simulink model "Comparison_between_Controllers"  (R2018b)
settings: Solver=VariableStepAuto  StartTime=0.0  StopTime=20000  FixedStep=1  RelTol=1e-3
undefined symbols (not defined in the file or in its folder): s
libraries: cstblocks x13, simulink x6, mpclib x3, slident x1
settings Model: Creator=Trips  LastModifiedBy=Trips

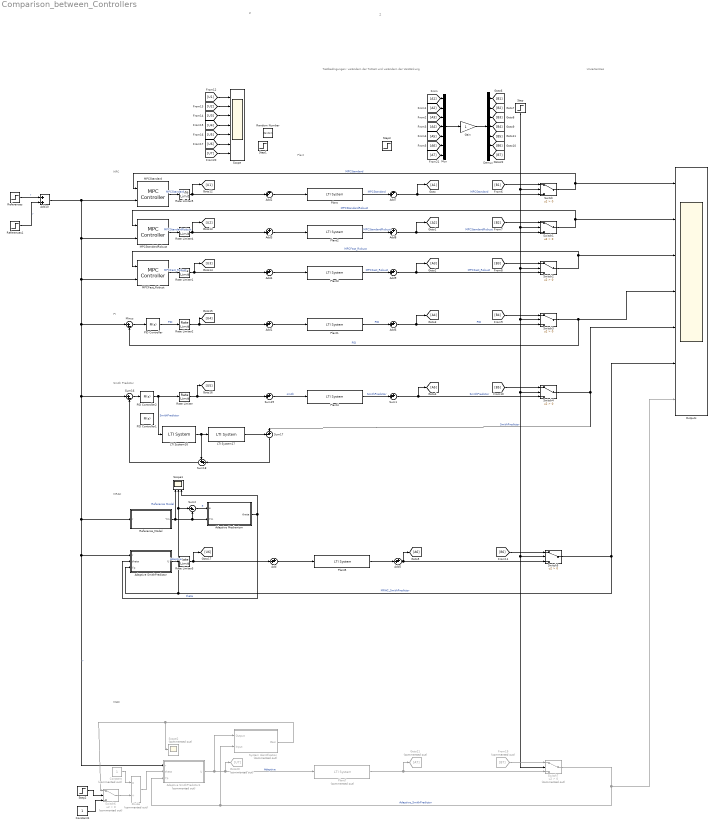
== system Comparison_between_Controllers ==
  note: MPC
  note: Testbedingungen: verändern der Totzeit und verändern der Verstärkung
  note: PI
  note: Smith Predictor
  note: Z
  note: Uncertainties
  note: Plant
  note: MRAC
  note: MIAC
  note: Z
  Adaptive Mechanism : Subsystem
  Adaptive SmithPredictor : Subsystem
  Adaptive SmithPredictor1 : Subsystem  Commented=on
  Add{,1..9} (10 alike) : Sum  Inputs=++|
  Add10 : Sum
  Constant : Constant  Commented=on
  Constant1 : Constant
  Demux : Demux  Outputs=7
  Divide : Product  Commented=on  Inputs=*/
  From19 : From  Commented=on  GotoTag=B7
  Gain : Gain
  Goto20 : Goto  Commented=on  GotoTag=U7
  Goto21 : Goto  Commented=on  GotoTag=A7
  LTI System16 : cstblocks/LTI System  sys=0.5/(700*s+1)  IC=[]
  LTI System17 : cstblocks/LTI System  sys=exp(-s*600)  IC=[]
  MPCFast_Robust : mpclib/MPC Controller  SCDEnableBlockLinearizationSpecification=on  mpcobj=mpc1_Faster_Robust  is_multiple=0  enable_value=0  return_u0=off  updateMPCinCallerWorkspace=on  md_inport=off  mv_inport=off  return_cost=off  return_mvseq=off  return_qpstatus=off  return_xseq=off  return_state=off  return_ovseq=off  state_inport=off  umin_inport=off  umax_inport=off  ymin_inport=off  ymax_inport=off  cc_inport=off  ywt_inport=off  uwt_inport=off  duwt_inport=off  rhoeps_inport=off  uref_inport=off  n_ts=70  n_p=15  n_mv=1  n_md=0  n_ud=0  n_mo=1  n_uo=0  BlockDataType=double  SampleTimeInherited=off  switch_inport=off
  MPCStandard : mpclib/MPC Controller  SCDEnableBlockLinearizationSpecification=on  mpcobj=mpc_Standard  is_multiple=0  enable_value=0  return_u0=off  updateMPCinCallerWorkspace=on  md_inport=off  mv_inport=off  return_cost=off  return_mvseq=off  return_qpstatus=off  return_xseq=off  return_state=off  return_ovseq=off  state_inport=off  umin_inport=off  umax_inport=off  ymin_inport=off  ymax_inport=off  cc_inport=off  ywt_inport=off  uwt_inport=off  duwt_inport=off  rhoeps_inport=off  uref_inport=off  n_ts=153  n_p=10  n_mv=1  n_md=0  n_ud=0  n_mo=1  n_uo=0  BlockDataType=double  SampleTimeInherited=off  switch_inport=off
  MPCStandardRobust : mpclib/MPC Controller  SCDEnableBlockLinearizationSpecification=on  mpcobj=mpc1_Standard_Robust  is_multiple=0  enable_value=0  return_u0=off  updateMPCinCallerWorkspace=on  md_inport=off  mv_inport=off  return_cost=off  return_mvseq=off  return_qpstatus=off  return_xseq=off  return_state=off  return_ovseq=off  state_inport=off  umin_inport=off  umax_inport=off  ymin_inport=off  ymax_inport=off  cc_inport=off  ywt_inport=off  uwt_inport=off  duwt_inport=off  rhoeps_inport=off  uref_inport=off  n_ts=153  n_p=10  n_mv=1  n_md=0  n_ud=0  n_mo=1  n_uo=0  BlockDataType=double  SampleTimeInherited=off  switch_inport=off
  Minus : Sum  Inputs=|+-
  Mux : Mux  Inputs=7
  Outputs : Scope  NumInputPorts=7
  PID Controller : simulink/Continuous/PID Controller  Controller=PI  Form=Parallel  TimeDomain=Continuous-time  SampleTime=-1  IntegratorMethod=Forward Euler  FilterMethod=Forward Euler  ControllerParametersSource=internal  P=1.81017492228937  I=0.00195107565412744  D=118.272348286844  UseFilter=on  N=0.00420306193364532  TunerSelectOption=Transfer Function Based (PID Tuner App)  InitialConditionSource=internal  InitialConditionForIntegrator=0  InitialConditionForFilter=0  DifferentiatorICPrevScaledInput=0  ExternalReset=none  TrackingMode=off  Kt=1  LimitOutput=on  UpperSaturationLimit=100  LowerSaturationLimit=0  LinearizeAsGain=on  AntiWindupMode=none  Kb=1  POutMin=[]  POutMax=[]  IOutMin=[]  IOutMax=[]  DOutMin=[]  DOutMax=[]  NOutMin=[]  NOutMax=[]  SumOutMin=[]  SumOutMax=[]  SaturationOutMin=[]  SaturationOutMax=[]  PParamMin=[]  PParamMax=[]  IParamMin=[]  IParamMax=[]  DParamMin=[]  DParamMax=[]  NParamMin=[]  NParamMax=[]  KbParamMin=[]  KbParamMax=[]  KtParamMin=[]  KtParamMax=[]  KbOutMin=[]  KbOutMax=[]  KtOutMin=[]  KtOutMax=[]  IntegratorOutMin=[]  IntegratorOutMax=[]  FilterOutMin=[]  FilterOutMax=[]  SumI1OutMin=[]  SumI1OutMax=[]  SumI2OutMin=[]  SumI2OutMax=[]  SumI3OutMin=[]  SumI3OutMax=[]  SumI4OutMin=[]  SumI4OutMax=[]  SumDOutMin=[]  SumDOutMax=[]  DifferentiatorOutMin=[]  DifferentiatorOutMax=[]  FilterDiffOutCoefMin=[]  FilterDiffOutCoefMax=[]  ReciprocalOutMin=[]  ReciprocalOutMax=[]  SumDenOutMin=[]  SumDenOutMax=[]  SumNumOutMin=[]  SumNumOutMax=[]  DivideOutMin=[]  DivideOutMax=[]  IntegratorContinuousStateAttributes=''  IntegratorStateMustResolveToSignalObject=off  IntegratorRTWStateStorageClass=Auto  FilterContinuousStateAttributes=''  FilterStateMustResolveToSignalObject=off  FilterRTWStateStorageClass=Auto  ParallelPVariant=InternalParameters  IdealPVariant=Disabled  IVariant=InternalParameters  DVariant=Disabled  IntegratorVariant=Continuous  SatVariant=Enabled  AWVariant=Passthrough  PCopyVariant=Disabled  TRVariant=Disabled  FdbkBlocksVariant=Forward  IdealPFdbkVariant=Disabled  SatFdbkVariant=Disabled  DerivativeFilterVariant=Disabled  NVariant=Disabled  NCopyVariant=Disabled_SignalSpec  FilterICVariant=Disabled  IntegratorICVariant=InternalICs  ExternalResetVariant=Disabled  TRSumVariant=Passthrough  SumFdbkVariant=Disabled  SumVariant=Sum_PI
  PID Controller1 : simulink/Continuous/PID Controller  Controller=PI  Form=Parallel  TimeDomain=Continuous-time  SampleTime=-1  IntegratorMethod=Forward Euler  FilterMethod=Forward Euler  ControllerParametersSource=internal  P=2.08480938092905  I=0.0089383224092643  D=118.272348286844  UseFilter=on  N=0.00420306193364532  TunerSelectOption=Transfer Function Based (PID Tuner App)  InitialConditionSource=internal  InitialConditionForIntegrator=0  InitialConditionForFilter=0  DifferentiatorICPrevScaledInput=0  ExternalReset=none  TrackingMode=off  Kt=1  LimitOutput=on  UpperSaturationLimit=100  LowerSaturationLimit=0  LinearizeAsGain=on  AntiWindupMode=none  Kb=1  POutMin=[]  POutMax=[]  IOutMin=[]  IOutMax=[]  DOutMin=[]  DOutMax=[]  NOutMin=[]  NOutMax=[]  SumOutMin=[]  SumOutMax=[]  SaturationOutMin=[]  SaturationOutMax=[]  PParamMin=[]  PParamMax=[]  IParamMin=[]  IParamMax=[]  DParamMin=[]  DParamMax=[]  NParamMin=[]  NParamMax=[]  KbParamMin=[]  KbParamMax=[]  KtParamMin=[]  KtParamMax=[]  KbOutMin=[]  KbOutMax=[]  KtOutMin=[]  KtOutMax=[]  IntegratorOutMin=[]  IntegratorOutMax=[]  FilterOutMin=[]  FilterOutMax=[]  SumI1OutMin=[]  SumI1OutMax=[]  SumI2OutMin=[]  SumI2OutMax=[]  SumI3OutMin=[]  SumI3OutMax=[]  SumI4OutMin=[]  SumI4OutMax=[]  SumDOutMin=[]  SumDOutMax=[]  DifferentiatorOutMin=[]  DifferentiatorOutMax=[]  FilterDiffOutCoefMin=[]  FilterDiffOutCoefMax=[]  ReciprocalOutMin=[]  ReciprocalOutMax=[]  SumDenOutMin=[]  SumDenOutMax=[]  SumNumOutMin=[]  SumNumOutMax=[]  DivideOutMin=[]  DivideOutMax=[]  IntegratorContinuousStateAttributes=''  IntegratorStateMustResolveToSignalObject=off  IntegratorRTWStateStorageClass=Auto  FilterContinuousStateAttributes=''  FilterStateMustResolveToSignalObject=off  FilterRTWStateStorageClass=Auto  ParallelPVariant=InternalParameters  IdealPVariant=Disabled  IVariant=InternalParameters  DVariant=Disabled  IntegratorVariant=Continuous  SatVariant=Enabled  AWVariant=Passthrough  PCopyVariant=Disabled  TRVariant=Disabled  FdbkBlocksVariant=Forward  IdealPFdbkVariant=Disabled  SatFdbkVariant=Disabled  DerivativeFilterVariant=Disabled  NVariant=Disabled  NCopyVariant=Disabled_SignalSpec  FilterICVariant=Disabled  IntegratorICVariant=InternalICs  ExternalResetVariant=Disabled  TRSumVariant=Passthrough  SumFdbkVariant=Disabled  SumVariant=Sum_PI
  PID Controller2 : simulink/Continuous/PID Controller  Controller=PI  Form=Parallel  TimeDomain=Continuous-time  SampleTime=-1  IntegratorMethod=Forward Euler  FilterMethod=Forward Euler  ControllerParametersSource=internal  P=3.04732259067536  I=0.00445689106465138  D=118.272348286844  UseFilter=on  N=0.00420306193364532  TunerSelectOption=Transfer Function Based (PID Tuner App)  InitialConditionSource=internal  InitialConditionForIntegrator=0  InitialConditionForFilter=0  DifferentiatorICPrevScaledInput=0  ExternalReset=none  TrackingMode=off  Kt=1  LimitOutput=on  UpperSaturationLimit=100  LowerSaturationLimit=0  LinearizeAsGain=on  AntiWindupMode=none  Kb=1  POutMin=[]  POutMax=[]  IOutMin=[]  IOutMax=[]  DOutMin=[]  DOutMax=[]  NOutMin=[]  NOutMax=[]  SumOutMin=[]  SumOutMax=[]  SaturationOutMin=[]  SaturationOutMax=[]  PParamMin=[]  PParamMax=[]  IParamMin=[]  IParamMax=[]  DParamMin=[]  DParamMax=[]  NParamMin=[]  NParamMax=[]  KbParamMin=[]  KbParamMax=[]  KtParamMin=[]  KtParamMax=[]  KbOutMin=[]  KbOutMax=[]  KtOutMin=[]  KtOutMax=[]  IntegratorOutMin=[]  IntegratorOutMax=[]  FilterOutMin=[]  FilterOutMax=[]  SumI1OutMin=[]  SumI1OutMax=[]  SumI2OutMin=[]  SumI2OutMax=[]  SumI3OutMin=[]  SumI3OutMax=[]  SumI4OutMin=[]  SumI4OutMax=[]  SumDOutMin=[]  SumDOutMax=[]  DifferentiatorOutMin=[]  DifferentiatorOutMax=[]  FilterDiffOutCoefMin=[]  FilterDiffOutCoefMax=[]  ReciprocalOutMin=[]  ReciprocalOutMax=[]  SumDenOutMin=[]  SumDenOutMax=[]  SumNumOutMin=[]  SumNumOutMax=[]  DivideOutMin=[]  DivideOutMax=[]  IntegratorContinuousStateAttributes=''  IntegratorStateMustResolveToSignalObject=off  IntegratorRTWStateStorageClass=Auto  FilterContinuousStateAttributes=''  FilterStateMustResolveToSignalObject=off  FilterRTWStateStorageClass=Auto  ParallelPVariant=InternalParameters  IdealPVariant=Disabled  IVariant=InternalParameters  DVariant=Disabled  IntegratorVariant=Continuous  SatVariant=Enabled  AWVariant=Passthrough  PCopyVariant=Disabled  TRVariant=Disabled  FdbkBlocksVariant=Forward  IdealPFdbkVariant=Disabled  SatFdbkVariant=Disabled  DerivativeFilterVariant=Disabled  NVariant=Disabled  NCopyVariant=Disabled_SignalSpec  FilterICVariant=Disabled  IntegratorICVariant=InternalICs  ExternalResetVariant=Disabled  TRSumVariant=Passthrough  SumFdbkVariant=Disabled  SumVariant=Sum_PI
  Plant{,1..5} (6 alike) : cstblocks/LTI System  sys=0.5/(700*s+1)*exp(-s*600)  IC=[]
  Plant7 : cstblocks/LTI System  Commented=on  sys=0.5/(700*s+1)*exp(-s*600)  IC=[]
  Random Number : RandomNumber  Variance=2  SampleTime=1000
  Rate Limiter{,1..5} (6 alike) : RateLimiter  RisingSlewLimit=0.05  FallingSlewLimit=-0.05  SampleTimeMode=inherited
  Reference_Model : Subsystem
  References : Step
  References1 : Step  Time=12000  After=2
  Scope : Scope  NumInputPorts=7
  Scope1 : Scope  NumInputPorts=3
  Scope2 : Scope  Commented=on
  Step : Step  Time=0  SampleTime=0
  Step1 : Step  Time=4000  After=-1  SampleTime=0
  Step2 : Step  Time=800  SampleTime=0
  Step3 : Step  Time=7000  After=-1  SampleTime=0
  Sum1 : Sum  Inputs=++|
  Sum16 : Sum  Inputs=|+-
  Sum17 : Sum  Inputs=-+|
  Sum18 : Sum  Inputs=++|
  Sum19 : Sum  Inputs=++|
  Sum2 : Sum  Inputs=|+-
  Switch{,1..5} (6 alike) : Switch  Criteria=u2 > Threshold
  Switch6 : Switch  Commented=on  Criteria=u2 > Threshold
  Switch7 : Switch  Commented=on  Criteria=u2 > Threshold
  System Identification : Subsystem  Commented=on
  wires:
  MPCStandard/1 -> Rate Limiter5/1  "MPCStandard"
  Add2/1 -> Plant/1
  Switch/1 -> MPCStandard/1, Outputs/1  "MPCStandard"
  PID Controller/1 -> Rate Limiter2/1  "PID"
  Minus/1 -> PID Controller/1
  Switch3/1 -> Minus/2, Outputs/4  "PID"
  Add1/1 -> Plant1/1
  ? -> Add2/1, Sum19/1, Add/1, Add1/1, Add4/1, Add3/1
  MPCStandardRobust/1 -> Rate Limiter4/1  "MPCStandardRobust"
  Switch1/1 -> MPCStandardRobust/1, Outputs/2  "MPCStandardRobust"
  Add3/1 -> Plant2/1
  MPCFast_Robust/1 -> Rate Limiter1/1  "MPCFast_Robust"
  Switch2/1 -> MPCFast_Robust/1, Outputs/3  "MPCFast_Robust"
  Add4/1 -> Plant3/1
  Sum17/1 -> Sum18/2
  LTI System16/1 -> LTI System17/1, Sum18/1
  Sum18/1 -> Sum16/2
  LTI System17/1 -> Sum17/1
  PID Controller2/1 -> Rate Limiter/1, LTI System16/1  "SmithPredictor"
  Sum16/1 -> PID Controller2/1
  Sum19/1 -> Plant4/1  "smith"
  Add7/1 -> [A1], Switch/3  "MPCStandard"
  Add8/1 -> Switch1/3, [A2]  "MPCStandardRobust"
  Add9/1 -> Switch2/3, [A3]  "MPCFast_Robust"
  Add6/1 -> Switch3/3, [A4]  "PID"
  Sum1/1 -> Switch4/3, [A5]  "SmithPredictor"
  Demux/3 -> [B3]
  Demux/2 -> [B2]
  Demux/1 -> [B1]
  Step/1 -> Switch2/2, Switch3/2, Switch4/2, Switch5/2, Switch7/2, Switch1/2, Switch/2
  Switch4/1 -> Sum17/2, Outputs/5  "SmithPredictor"
  Rate Limiter/1 -> [U5], Sum19/2
  Rate Limiter1/1 -> [U3], Add4/2
  Reference_Model/1(Ym) -> Adaptive Mechanism/2(Ym), Sum2/2, Scope1/1  "Reference Model"
  Add5/1 -> [A6], Switch5/3
  Adaptive SmithPredictor/1(U) -> Rate Limiter3/1  "Adaptive"
  Add10/1 -> MPCStandard/2, MPCStandardRobust/2, MPCFast_Robust/2, Sum16/1, Reference_Model/1(r), Adaptive SmithPredictor1/1(r), Adaptive SmithPredictor/1(r), Minus/1  "r"
  Adaptive Mechanism/1(theta) -> Adaptive SmithPredictor/2(theta), Scope1/3  "theta"
  Add/1 -> Plant5/1
  Sum2/1 -> Adaptive Mechanism/1(e)  "e"
  Switch5/1 -> Adaptive SmithPredictor/3(Yp), Scope1/2, Sum2/1, Outputs/6  "MRAC_SmithPredictor"
  [B6] -> Switch5/1
  [A1] -> Mux/1
  [A2] -> Mux/2
  [A3] -> Mux/3
  [A4] -> Mux/4
  [A5] -> Mux/5
  [A6] -> Mux/6
  Demux/6 -> [B6]
  Demux/4 -> [B4]
  Demux/5 -> [B5]
  [B1] -> Switch/1
  [B2] -> Switch1/1
  [B3] -> Switch2/1
  [B4] -> Switch3/1
  [B5] -> Switch4/1
  Mux/1 -> Gain/1
  Gain/1 -> Demux/1
  [U1] -> Scope/1
  [U2] -> Scope/2
  [U3] -> Scope/3
  [U4] -> Scope/4
  [U5] -> Scope/5
  [U6] -> Scope/6
  Switch7/1 -> Outputs/7, System Identification/2(Input), Adaptive SmithPredictor1/3(Yp)  "Adaptive_SmithPredictor"
  Adaptive SmithPredictor1/1(U) -> System Identification/1(Output), Goto20/1, Plant7/1  "Adaptive"
  Plant7/1 -> Goto21/1, Switch7/3
  [U7] -> Scope/7
  [A7] -> Mux/7
  Demux/7 -> [B7]
  From19/1 -> Switch7/1
  Divide/1 -> Adaptive SmithPredictor1/2(theta)
  Constant1/1 -> Switch6/3
  Step2/1 -> Switch6/2
  System Identification/1(Gain) -> Switch6/1, Scope2/1
  Constant/1 -> Divide/1
  Switch6/1 -> Divide/2
  ? -> Add7/1, Sum1/1, Add5/1, Add6/1, Add9/1, Add8/1
  Plant5/1 -> Add5/2
  Plant4/1 -> Sum1/2  "SmithPredictor"
  Plant1/1 -> Add6/2  "PID"
  Plant3/1 -> Add9/2  "MPCFast_Robust"
  Plant2/1 -> Add8/2  "MPCStandardRobust"
  Plant/1 -> Add7/2  "MPCStandard"
  References/1 -> Add10/1  "r"
  References1/1 -> Add10/2  "r"
  Rate Limiter2/1 -> Add1/2, [U4]
  Rate Limiter3/1 -> [U6], Add/2
  Rate Limiter4/1 -> [U2], Add3/2
  Rate Limiter5/1 -> [U1], Add2/2

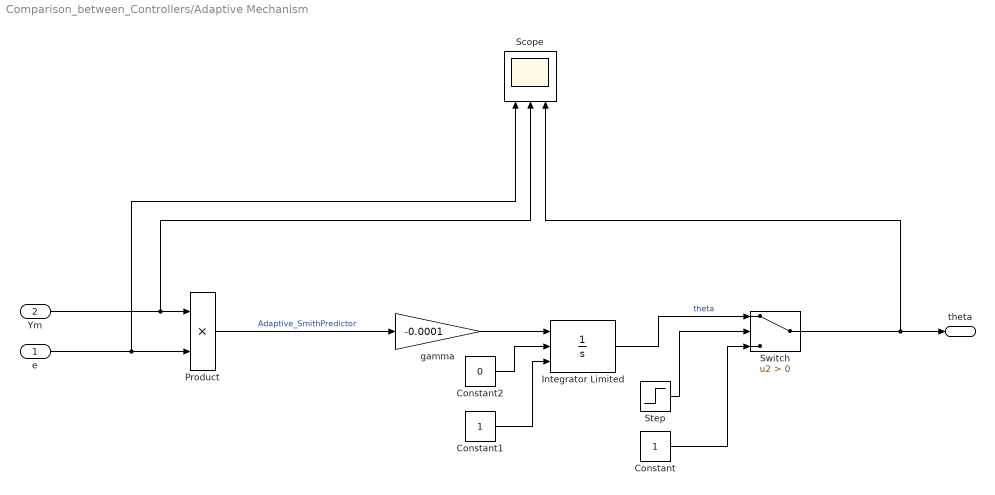
== system Comparison_between_Controllers/Adaptive Mechanism ==
  e : Inport
  Ym : Inport  Port=2
  Constant : Constant
  Constant1 : Constant
  Constant2 : Constant  Value=0
  Integrator Limited : Integrator  ExternalReset=rising  InitialConditionSource=external  InitialCondition=1  LimitOutput=on  UpperSaturationLimit=100  LowerSaturationLimit=-100
  Product : Product
  Scope : Scope  NumInputPorts=3
  Step : Step  Time=0  SampleTime=0
  Switch : Switch  Criteria=u2 > Threshold
  gamma : Gain  Gain=-0.0001
  theta : Outport
  wires:
  Switch/1 -> Scope/3, theta/1
  Ym/1 -> Scope/2, Product/1
  e/1 -> Scope/1, Product/2
  gamma/1 -> Integrator Limited/1
  Integrator Limited/1 -> Switch/1  "theta"
  Constant/1 -> Switch/3
  Step/1 -> Switch/2
  Constant1/1 -> Integrator Limited/3
  Constant2/1 -> Integrator Limited/2
  Product/1 -> gamma/1  "Adaptive_SmithPredictor"

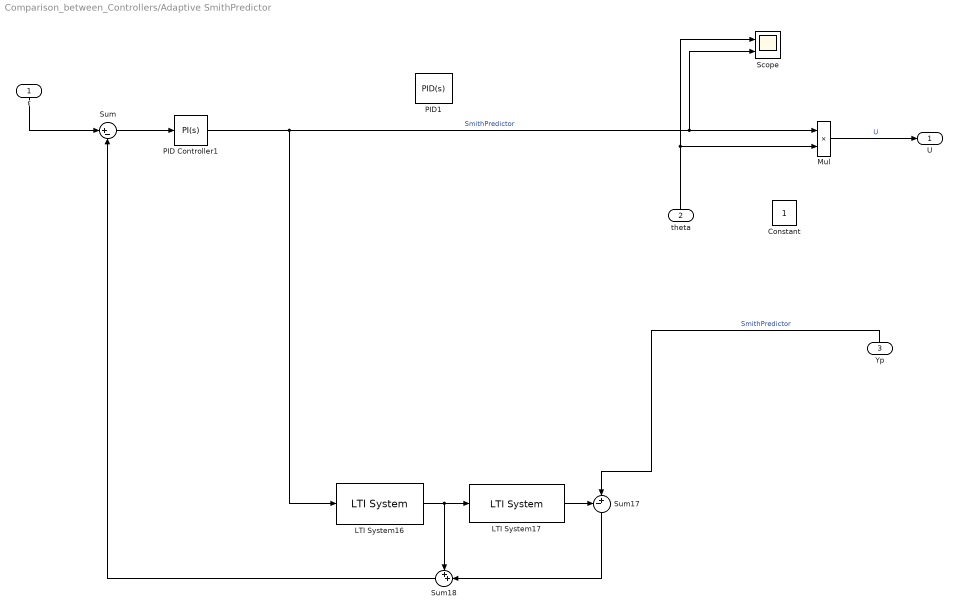
== system Comparison_between_Controllers/Adaptive SmithPredictor ==
  r : Inport
  theta : Inport  Port=2
  Yp : Inport  Port=3
  Constant : Constant
  LTI System16 : cstblocks/LTI System  sys=0.5/(700*s+1)  IC=[]
  LTI System17 : cstblocks/LTI System  sys=exp(-s*600)  IC=[]
  Mul : Product
  PID Controller1 : simulink/Continuous/PID Controller  Controller=PI  Form=Parallel  TimeDomain=Continuous-time  SampleTime=-1  IntegratorMethod=Forward Euler  FilterMethod=Forward Euler  ControllerParametersSource=internal  P=3.04732259067536  I=0.00445689106465138  D=118.272348286844  UseFilter=on  N=0.00420306193364532  TunerSelectOption=Transfer Function Based (PID Tuner App)  InitialConditionSource=internal  InitialConditionForIntegrator=0  InitialConditionForFilter=0  DifferentiatorICPrevScaledInput=0  ExternalReset=none  TrackingMode=off  Kt=1  LimitOutput=on  UpperSaturationLimit=100  LowerSaturationLimit=0  LinearizeAsGain=on  AntiWindupMode=none  Kb=1  POutMin=[]  POutMax=[]  IOutMin=[]  IOutMax=[]  DOutMin=[]  DOutMax=[]  NOutMin=[]  NOutMax=[]  SumOutMin=[]  SumOutMax=[]  SaturationOutMin=[]  SaturationOutMax=[]  PParamMin=[]  PParamMax=[]  IParamMin=[]  IParamMax=[]  DParamMin=[]  DParamMax=[]  NParamMin=[]  NParamMax=[]  KbParamMin=[]  KbParamMax=[]  KtParamMin=[]  KtParamMax=[]  KbOutMin=[]  KbOutMax=[]  KtOutMin=[]  KtOutMax=[]  IntegratorOutMin=[]  IntegratorOutMax=[]  FilterOutMin=[]  FilterOutMax=[]  SumI1OutMin=[]  SumI1OutMax=[]  SumI2OutMin=[]  SumI2OutMax=[]  SumI3OutMin=[]  SumI3OutMax=[]  SumI4OutMin=[]  SumI4OutMax=[]  SumDOutMin=[]  SumDOutMax=[]  DifferentiatorOutMin=[]  DifferentiatorOutMax=[]  FilterDiffOutCoefMin=[]  FilterDiffOutCoefMax=[]  ReciprocalOutMin=[]  ReciprocalOutMax=[]  SumDenOutMin=[]  SumDenOutMax=[]  SumNumOutMin=[]  SumNumOutMax=[]  DivideOutMin=[]  DivideOutMax=[]  IntegratorContinuousStateAttributes=''  IntegratorStateMustResolveToSignalObject=off  IntegratorRTWStateStorageClass=Auto  FilterContinuousStateAttributes=''  FilterStateMustResolveToSignalObject=off  FilterRTWStateStorageClass=Auto  ParallelPVariant=InternalParameters  IdealPVariant=Disabled  IVariant=InternalParameters  DVariant=Disabled  IntegratorVariant=Continuous  SatVariant=Enabled  AWVariant=Passthrough  PCopyVariant=Disabled  TRVariant=Disabled  FdbkBlocksVariant=Forward  IdealPFdbkVariant=Disabled  SatFdbkVariant=Disabled  DerivativeFilterVariant=Disabled  NVariant=Disabled  NCopyVariant=Disabled_SignalSpec  FilterICVariant=Disabled  IntegratorICVariant=InternalICs  ExternalResetVariant=Disabled  TRSumVariant=Passthrough  SumFdbkVariant=Disabled  SumVariant=Sum_PI
  PID1 : simulink/Continuous/PID Controller  Controller=PID  Form=Parallel  TimeDomain=Continuous-time  SampleTime=1  IntegratorMethod=Forward Euler  FilterMethod=Forward Euler  ControllerParametersSource=internal  P=30  I=100  D=0  UseFilter=on  N=100  TunerSelectOption=Transfer Function Based (PID Tuner App)  InitialConditionSource=internal  InitialConditionForIntegrator=0  InitialConditionForFilter=0  DifferentiatorICPrevScaledInput=0  ExternalReset=none  TrackingMode=off  Kt=1  LimitOutput=on  UpperSaturationLimit=600  LowerSaturationLimit=-600  LinearizeAsGain=on  AntiWindupMode=clamping  Kb=1  POutMin=[]  POutMax=[]  IOutMin=[]  IOutMax=[]  DOutMin=[]  DOutMax=[]  NOutMin=[]  NOutMax=[]  SumOutMin=[]  SumOutMax=[]  SaturationOutMin=[]  SaturationOutMax=[]  PParamMin=[]  PParamMax=[]  IParamMin=[]  IParamMax=[]  DParamMin=[]  DParamMax=[]  NParamMin=[]  NParamMax=[]  KbParamMin=[]  KbParamMax=[]  KtParamMin=[]  KtParamMax=[]  KbOutMin=[]  KbOutMax=[]  KtOutMin=[]  KtOutMax=[]  IntegratorOutMin=[]  IntegratorOutMax=[]  FilterOutMin=[]  FilterOutMax=[]  SumI1OutMin=[]  SumI1OutMax=[]  SumI2OutMin=[]  SumI2OutMax=[]  SumI3OutMin=[]  SumI3OutMax=[]  SumI4OutMin=[]  SumI4OutMax=[]  SumDOutMin=[]  SumDOutMax=[]  DifferentiatorOutMin=[]  DifferentiatorOutMax=[]  FilterDiffOutCoefMin=[]  FilterDiffOutCoefMax=[]  ReciprocalOutMin=[]  ReciprocalOutMax=[]  SumDenOutMin=[]  SumDenOutMax=[]  SumNumOutMin=[]  SumNumOutMax=[]  DivideOutMin=[]  DivideOutMax=[]  IntegratorContinuousStateAttributes=''  IntegratorStateMustResolveToSignalObject=off  IntegratorRTWStateStorageClass=Auto  FilterContinuousStateAttributes=''  FilterStateMustResolveToSignalObject=off  FilterRTWStateStorageClass=Auto  ParallelPVariant=InternalParameters  IdealPVariant=Disabled  IVariant=InternalParameters  DVariant=InternalParameters  IntegratorVariant=Continuous  SatVariant=Enabled  AWVariant=ContClampingParallel  PCopyVariant=Disabled  TRVariant=Disabled  FdbkBlocksVariant=Forward  IdealPFdbkVariant=Disabled  SatFdbkVariant=Disabled  DerivativeFilterVariant=ContFilter  NVariant=InternalParameters  NCopyVariant=Disabled  FilterICVariant=InternalICsFilter  IntegratorICVariant=InternalICs  ExternalResetVariant=Disabled  TRSumVariant=Passthrough  SumFdbkVariant=Disabled  SumVariant=Sum_PID
  Scope : Scope  NumInputPorts=2
  Sum : Sum  Inputs=|+-
  Sum17 : Sum  Inputs=-+|
  Sum18 : Sum  Inputs=++|
  U : Outport
  wires:
  r/1 -> Sum/1
  Sum/1 -> PID Controller1/1
  Mul/1 -> U/1  "U"
  PID Controller1/1 -> LTI System16/1, Scope/2, Mul/1  "SmithPredictor"
  Yp/1 -> Sum17/2  "SmithPredictor"
  LTI System16/1 -> LTI System17/1, Sum18/1
  Sum18/1 -> Sum/2
  LTI System17/1 -> Sum17/1
  Sum17/1 -> Sum18/2
  theta/1 -> Mul/2, Scope/1

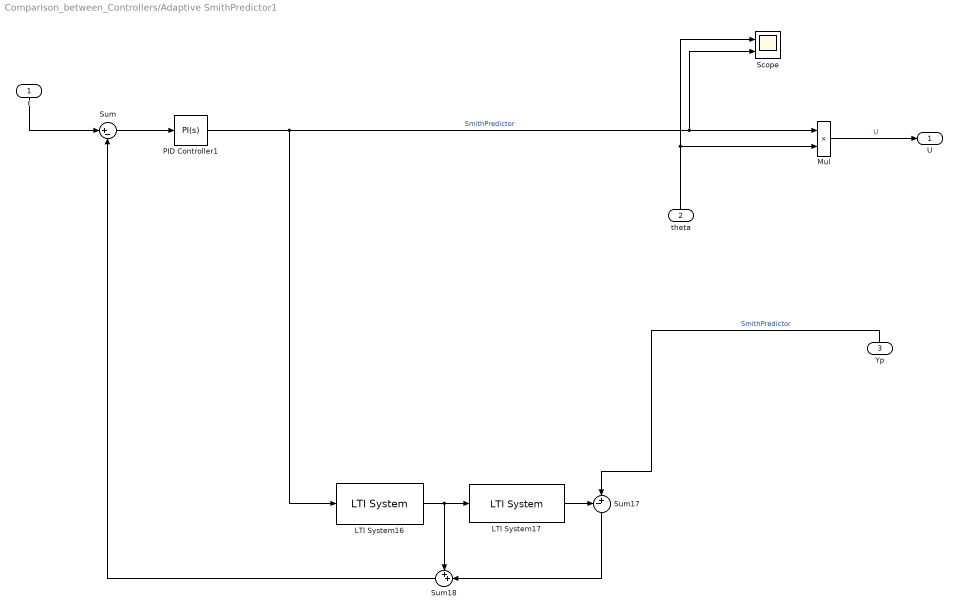
== system Comparison_between_Controllers/Adaptive SmithPredictor1 ==
  r : Inport
  theta : Inport  Port=2
  Yp : Inport  Port=3
  LTI System16 : cstblocks/LTI System  sys=0.5/(700*s+1)  IC=[]
  LTI System17 : cstblocks/LTI System  sys=exp(-s*600)  IC=[]
  Mul : Product
  PID Controller1 : simulink/Continuous/PID Controller  Controller=PI  Form=Parallel  TimeDomain=Continuous-time  SampleTime=-1  IntegratorMethod=Forward Euler  FilterMethod=Forward Euler  ControllerParametersSource=internal  P=3.04732259067536  I=0.00445689106465138  D=118.272348286844  UseFilter=on  N=0.00420306193364532  TunerSelectOption=Transfer Function Based (PID Tuner App)  InitialConditionSource=internal  InitialConditionForIntegrator=0  InitialConditionForFilter=0  DifferentiatorICPrevScaledInput=0  ExternalReset=none  TrackingMode=off  Kt=1  LimitOutput=on  UpperSaturationLimit=100  LowerSaturationLimit=0  LinearizeAsGain=on  AntiWindupMode=none  Kb=1  POutMin=[]  POutMax=[]  IOutMin=[]  IOutMax=[]  DOutMin=[]  DOutMax=[]  NOutMin=[]  NOutMax=[]  SumOutMin=[]  SumOutMax=[]  SaturationOutMin=[]  SaturationOutMax=[]  PParamMin=[]  PParamMax=[]  IParamMin=[]  IParamMax=[]  DParamMin=[]  DParamMax=[]  NParamMin=[]  NParamMax=[]  KbParamMin=[]  KbParamMax=[]  KtParamMin=[]  KtParamMax=[]  KbOutMin=[]  KbOutMax=[]  KtOutMin=[]  KtOutMax=[]  IntegratorOutMin=[]  IntegratorOutMax=[]  FilterOutMin=[]  FilterOutMax=[]  SumI1OutMin=[]  SumI1OutMax=[]  SumI2OutMin=[]  SumI2OutMax=[]  SumI3OutMin=[]  SumI3OutMax=[]  SumI4OutMin=[]  SumI4OutMax=[]  SumDOutMin=[]  SumDOutMax=[]  DifferentiatorOutMin=[]  DifferentiatorOutMax=[]  FilterDiffOutCoefMin=[]  FilterDiffOutCoefMax=[]  ReciprocalOutMin=[]  ReciprocalOutMax=[]  SumDenOutMin=[]  SumDenOutMax=[]  SumNumOutMin=[]  SumNumOutMax=[]  DivideOutMin=[]  DivideOutMax=[]  IntegratorContinuousStateAttributes=''  IntegratorStateMustResolveToSignalObject=off  IntegratorRTWStateStorageClass=Auto  FilterContinuousStateAttributes=''  FilterStateMustResolveToSignalObject=off  FilterRTWStateStorageClass=Auto  ParallelPVariant=InternalParameters  IdealPVariant=Disabled  IVariant=InternalParameters  DVariant=Disabled  IntegratorVariant=Continuous  SatVariant=Enabled  AWVariant=Passthrough  PCopyVariant=Disabled  TRVariant=Disabled  FdbkBlocksVariant=Forward  IdealPFdbkVariant=Disabled  SatFdbkVariant=Disabled  DerivativeFilterVariant=Disabled  NVariant=Disabled  NCopyVariant=Disabled_SignalSpec  FilterICVariant=Disabled  IntegratorICVariant=InternalICs  ExternalResetVariant=Disabled  TRSumVariant=Passthrough  SumFdbkVariant=Disabled  SumVariant=Sum_PI
  Scope : Scope  NumInputPorts=2
  Sum : Sum  Inputs=|+-
  Sum17 : Sum  Inputs=-+|
  Sum18 : Sum  Inputs=++|
  U : Outport
  wires:
  r/1 -> Sum/1
  Sum/1 -> PID Controller1/1
  Mul/1 -> U/1  "U"
  PID Controller1/1 -> LTI System16/1, Scope/2, Mul/1  "SmithPredictor"
  Yp/1 -> Sum17/2  "SmithPredictor"
  LTI System16/1 -> LTI System17/1, Sum18/1
  Sum18/1 -> Sum/2
  LTI System17/1 -> Sum17/1
  Sum17/1 -> Sum18/2
  theta/1 -> Mul/2, Scope/1

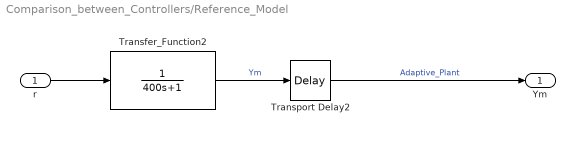
== system Comparison_between_Controllers/Reference_Model ==
  r : Inport
  Transfer_Function2 : TransferFcn  Denominator=[400 1]
  Transport Delay2 : TransportDelay  DelayTime=600
  Ym : Outport
  wires:
  Transfer_Function2/1 -> Transport Delay2/1  "Ym"
  r/1 -> Transfer_Function2/1
  Transport Delay2/1 -> Ym/1  "Adaptive_Plant"

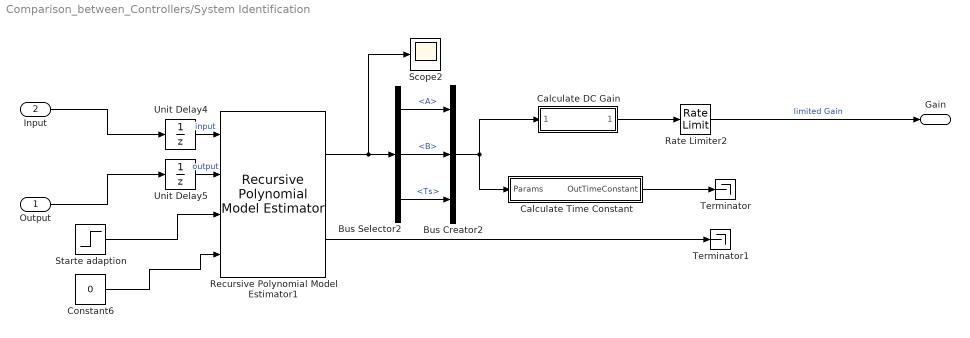
== system Comparison_between_Controllers/System Identification ==
  Output : Inport
  Input : Inport  Port=2
  Bus Creator2 : BusCreator  Inputs=3
  Bus Selector2 : BusSelector  OutputSignals=A,B,Ts
  Calculate DC Gain : Subsystem
  Calculate Time Constant : Subsystem
  Constant6 : Constant  Value=0
  Rate Limiter2 : RateLimiter  SampleTimeMode=inherited
  Recursive Polynomial Model Estimator1 : slident/Estimators/Recursive Polynomial Model Estimator  ModelStructure=ARX  InitialEstimateSource=None  A0=1  B0=1  C0=1  D0=1  F0=1  nk=1  P0=1  InitialInputs=0  InitialOutputs=0  History=Infinite  WindowLength=5  EstimationMethod=Kalman Filter  AdaptationParameter=0.01  HasTimeVaryingAdaptationParameter=off  NormalizationBias=eps  OutputError=on  OutputP=off  AddEnablePort=on  ExternalReset=Rising  InputProcessing=Sample-based  Ts=1
      settings: SourceProductName=System Identification Toolbox  SourceProductBaseCode=ID
  Scope2 : Scope
  Starte adaption : Step  Time=0  SampleTime=0.1
  Terminator : Terminator
  Terminator1 : Terminator
  Unit Delay4 : UnitDelay  InitialCondition=[0]  SampleTime=0.1
  Unit Delay5 : UnitDelay  SampleTime=0.1
  Gain : Outport
  wires:
  Bus Selector2/1 -> Bus Creator2/1  "<A>"
  Recursive Polynomial Model Estimator1/1 -> Scope2/1, Bus Selector2/1
  Bus Selector2/3 -> Bus Creator2/3  "<Ts>"
  Bus Selector2/2 -> Bus Creator2/2  "<B>"
  Bus Creator2/1 -> Calculate DC Gain/1(Params), Calculate Time Constant/1(Params)
  Recursive Polynomial Model Estimator1/2 -> Terminator1/1
  Rate Limiter2/1 -> Gain/1  "limited Gain"
  Calculate Time Constant/1("OutTimeConstant ") -> Terminator/1
  Calculate DC Gain/1(DCGain) -> Rate Limiter2/1
  Constant6/1 -> Recursive Polynomial Model Estimator1/4
  Unit Delay4/1 -> Recursive Polynomial Model Estimator1/1  "input"
  Unit Delay5/1 -> Recursive Polynomial Model Estimator1/2  "output"
  Input/1 -> Unit Delay4/1
  Output/1 -> Unit Delay5/1
  Starte adaption/1 -> Recursive Polynomial Model Estimator1/3

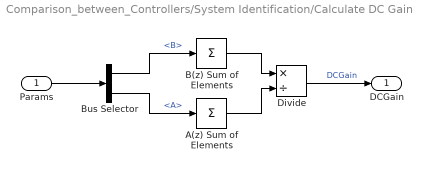
== system Comparison_between_Controllers/System Identification/Calculate DC Gain ==
  Params : Inport
  A(z) Sum of Elements : Sum  Inputs=+
  B(z) Sum of Elements : Sum  Inputs=+
  Bus Selector : BusSelector  OutputSignals=B,A
  Divide : Product  Inputs=*/
  DCGain : Outport
  wires:
  A(z) Sum of Elements/1 -> Divide/2
  B(z) Sum of Elements/1 -> Divide/1
  Params/1 -> Bus Selector/1
  Bus Selector/1 -> B(z) Sum of Elements/1  "<B>"
  Bus Selector/2 -> A(z) Sum of Elements/1  "<A>"
  Divide/1 -> DCGain/1  "DCGain"

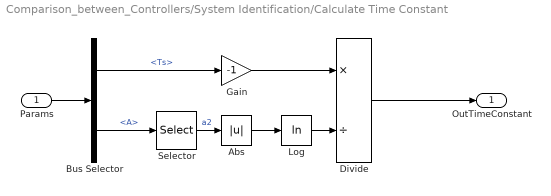
== system Comparison_between_Controllers/System Identification/Calculate Time Constant ==
  Params : Inport
  Abs : Abs
  Bus Selector : BusSelector  OutputSignals=Ts,A
  Divide : Product  Inputs=*/
  Gain : Gain  Gain=-1
  Log : Math  Operator=log  SaturateOnIntegerOverflow=on
  Selector : Selector  InputPortWidth=2  IndexOptions=Starting index (dialog)  Indices=[2]  OutputSizes=1
  "OutTimeConstant " : Outport
  wires:
  Params/1 -> Bus Selector/1
  Bus Selector/1 -> Gain/1  "<Ts>"
  Bus Selector/2 -> Selector/1  "<A>"
  Selector/1 -> Abs/1  "a2"
  Gain/1 -> Divide/1
  Log/1 -> Divide/2
  Divide/1 -> "OutTimeConstant "/1
  Abs/1 -> Log/1
